simulink model "plant"  (R2023a)
settings: Solver=ode4  StartTime=0.0  StopTime=t_duration  FixedStep=dt  RelTol=1e-3
undefined symbols (not defined in the file): deputy1, deputy2
settings Model: Creator=ndelurgio  LastModifiedBy=ndelurgio
settings DebuggingCC: ModelReferenceExtraNoncontSigs=none

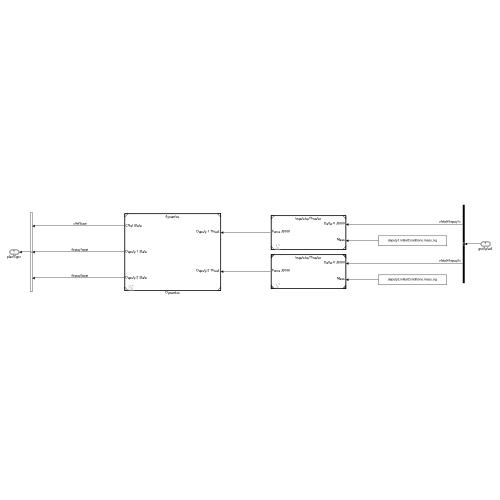
[thumbnail: Simulink's stored preview of the top-level diagram]
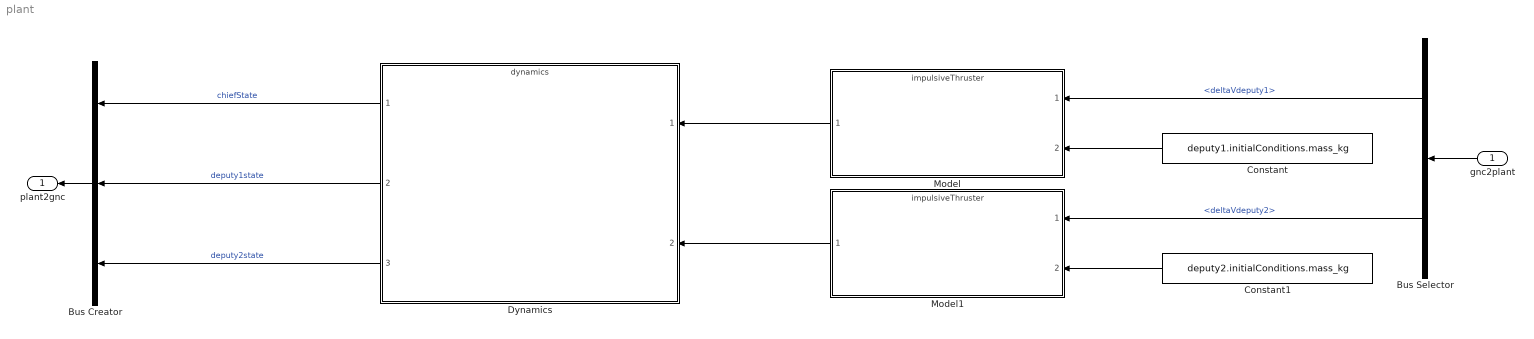
== system plant ==
  gnc2plant : Inport  OutDataTypeStr=Bus: gnc2plant
  Bus Creator : BusCreator  Inputs=3  OutDataTypeStr=Bus: plant2gnc  NonVirtualBus=on
      settings: InheritFromInputs=off
  Bus Selector : BusSelector  OutputSignals=deltaVdeputy1,deltaVdeputy2
  Constant : Constant  Value=deputy1.initialConditions.mass_kg
  Constant1 : Constant  Value=deputy2.initialConditions.mass_kg
  Dynamics : ModelReference  ModelNameDialog=dynamics  SimulationMode=Normal  ModelReferenceVersion=1.39
  Model : ModelReference  ModelNameDialog=impulsiveThruster  SimulationMode=Normal  ModelReferenceVersion=1.5
  Model1 : ModelReference  ModelNameDialog=impulsiveThruster  SimulationMode=Normal  ModelReferenceVersion=1.5
  plant2gnc : Outport  OutDataTypeStr=Bus: plant2gnc  BusOutputAsStruct=on
  wires:
  Dynamics/2 -> Bus Creator/2  "deputy1state"
  Dynamics/1 -> Bus Creator/1  "chiefState"
  Bus Creator/1 -> plant2gnc/1
  Model/1 -> Dynamics/1
  Bus Selector/1 -> Model/1  "<deltaVdeputy1>"
  Constant/1 -> Model/2
  Constant1/1 -> Model1/2
  Bus Selector/2 -> Model1/1  "<deltaVdeputy2>"
  Model1/1 -> Dynamics/2
  Dynamics/3 -> Bus Creator/3  "deputy2state"
  gnc2plant/1 -> Bus Selector/1
